simulink model "model_bf_margin"  (Simulink 7.0)
settings: Solver=ode45  StartTime=0.0  StopTime=10.0  RelTol=1e-3
libraries: cstblocks x2
settings Model: Creator=fromion  LastModifiedBy=vfromion  ExtModeTrigMode=oneshot  ExtModeArmWhenConnect=off  ExtModeAutoUpdateStatusClock=off
settings DataIOCC: LimitDataPoints=off
settings OptimizationCC: BlockReduction=off  BooleanDataType=off
settings DebuggingCC: SaveWithParameterizedLinksMsg=none  SignalResolutionControl=TryResolveAllWithWarning  SolverPrmCheckMsg=none  MultiTaskDSMMsg=warning  MultiTaskCondExecSysMsg=none  StrictBusMsg=None
settings HardwareCC: TargetUnknown=on
settings RTWCC: IncludeERTFirstTime=on
settings STFCustomTargetCC: GenFloatMathFcnCalls=ANSI_C  ModelReferenceCompliant=off  SystemTargetFile=grt.tlc

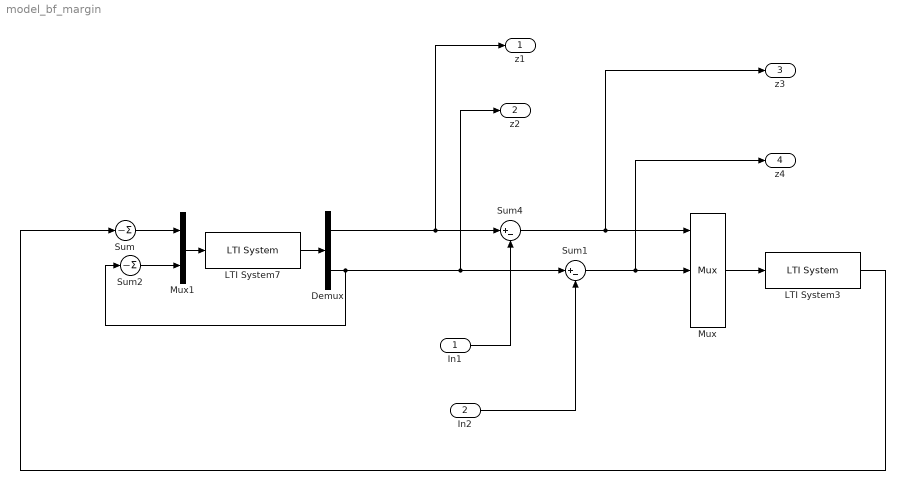
== system model_bf_margin ==
  In1 : Inport
  In2 : Inport  Port=2
  Demux : Demux  Outputs=2
  LTI System3 : cstblocks/LTI System  SystemSampleTime=-1  sys=sys_bo_ss  IC=0
  LTI System7 : cstblocks/LTI System  SystemSampleTime=-1  sys=K_hinf_ss  IC=0
  Mux : Mux  Inputs=3
  Mux1 : Mux  Inputs=2
  Sum : Sum  Inputs=-  SaturateOnIntegerOverflow=on  InputSameDT=on
  Sum1 : Sum  Inputs=|+-  SaturateOnIntegerOverflow=on  InputSameDT=on
  Sum2 : Sum  Inputs=-  SaturateOnIntegerOverflow=on  InputSameDT=on
  Sum4 : Sum  Inputs=|+-  SaturateOnIntegerOverflow=on  InputSameDT=on
  z1 : Outport
  z2 : Outport  Port=2
  z3 : Outport  Port=3
  z4 : Outport  Port=4
  wires:
  Sum/1 -> Mux1/1
  In1/1 -> Sum4/2
  LTI System3/1 -> Sum/1
  Sum4/1 -> Mux/1, z3/1
  Demux/2 -> Sum2/1, Sum1/1, z2/1
  Sum1/1 -> Mux/2, z4/1
  In2/1 -> Sum1/2
  Sum2/1 -> Mux1/2
  Mux/1 -> LTI System3/1
  Demux/1 -> Sum4/1, z1/1
  Mux1/1 -> LTI System7/1
  LTI System7/1 -> Demux/1
